simulink model "model_chirp_control_conMR_Bingham"  (R2016a)
settings: Solver=ode4  StartTime=0.0  StopTime=t_final2  FixedStep=tsam  RelTol=1e-3
values from neighbouring files (symbols this model uses):
  I1 = 0.01    [Run_MdE_Research_Report_con_MR_damper.m]
  kt = ((2*pi*ft)^2)*mt    [Run_MdE_Research_Report.m]    (also in Run_MdE_Research_Report_con_MR_damper.m; my_script.m)
  mt = mu*m1    (= 0.02)    [Run_MdE_Research_Report.m]    (also in Run_MdE_Research_Report_con_MR_damper.m = 40; my_script.m)
  sat = 50    [Run_MdE_Research_Report_con_MR_damper.m]
undefined symbols (not defined in the file or in its folder): D_Gs, N_Gs, ndata2, t_final2, tsam
libraries: simulink x1
settings Model: Creator=user  LastModifiedBy=usuario
settings DataIOCC: LimitDataPoints=on  SaveFormat=Array  SignalLoggingSaveFormat=ModelDataLogs  SignalLoggingName=sigsOut
settings OptimizationCC: InitFltsAndDblsToZero=on
settings DebuggingCC: SaveWithParameterizedLinksMsg=none  UnderspecifiedInitializationDetection=Classic  MergeDetectMultiDrivingBlocksExec=none  SignalResolutionControl=TryResolveAllWithWarning  MultiTaskDSMMsg=warning  MultiTaskCondExecSysMsg=none  FcnCallInpInsideContextMsg=EnableAllAsWarning
settings HardwareCC: ProdBitPerPointer=32  ProdLargestAtomicFloat=None  ProdIntDivRoundTo=Undefined  ProdEndianess=Unspecified  ProdWordSize=32  ProdHWDeviceType=32-bit Generic  TargetBitPerPointer=64  TargetLongLongMode=on  TargetIntDivRoundTo=Zero  TargetEndianess=LittleEndian  TargetWordSize=64  TargetHWDeviceType=MATLAB Host  ProdEqTarget=off
settings ModelReferenceCC: PropagateSignalLabelsOutOfModel=off
settings GRTTargetCC: TargetFcnLib=ansi_tfl_tmw.mat  CombineOutputUpdateFcns=off  GRTInterface=on
settings ConfigComp: CovModelRefEnable=Off  CovSFcnEnable=off

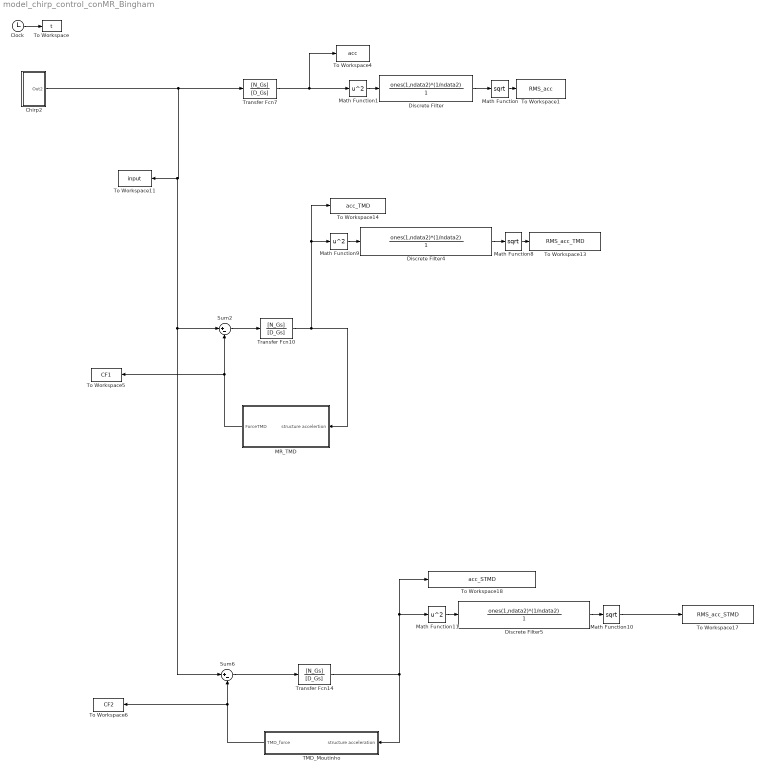
== system model_chirp_control_conMR_Bingham ==
  Chirp2 : Subsystem
  Clock : Clock
  Discrete Filter : DiscreteFilter  Numerator=ones(1,ndata2)*(1/ndata2)  Denominator=1  SampleTime=tsam
  Discrete Filter4 : DiscreteFilter  Numerator=ones(1,ndata2)*(1/ndata2)  Denominator=1  SampleTime=tsam
  Discrete Filter5 : DiscreteFilter  Numerator=ones(1,ndata2)*(1/ndata2)  Denominator=1  SampleTime=tsam
  MR_TMD : Subsystem
  Math Function : Math  Operator=sqrt  SampleTime=tsam  SaturateOnIntegerOverflow=on
  Math Function1 : Math  Operator=square  SampleTime=tsam  SaturateOnIntegerOverflow=on
  Math Function10 : Math  Operator=sqrt  SampleTime=tsam  SaturateOnIntegerOverflow=on
  Math Function11 : Math  Operator=square  SampleTime=tsam  SaturateOnIntegerOverflow=on
  Math Function8 : Math  Operator=sqrt  SampleTime=tsam  SaturateOnIntegerOverflow=on
  Math Function9 : Math  Operator=square  SampleTime=tsam  SaturateOnIntegerOverflow=on
  Sum2 : Sum  Inputs=|+-
  Sum6 : Sum  Inputs=|+-
  TMD_Moutinho : Subsystem
  To Workspace : ToWorkspace  VariableName=t  SampleTime=tsam
  To Workspace1 : ToWorkspace  VariableName=RMS_acc  SampleTime=tsam
  To Workspace11 : ToWorkspace  VariableName=input  SampleTime=tsam
  To Workspace13 : ToWorkspace  VariableName=RMS_acc_TMD  SampleTime=tsam
  To Workspace14 : ToWorkspace  VariableName=acc_TMD  SampleTime=tsam
  To Workspace17 : ToWorkspace  VariableName=RMS_acc_STMD  SampleTime=tsam
  To Workspace18 : ToWorkspace  VariableName=acc_STMD  SampleTime=tsam
  To Workspace4 : ToWorkspace  VariableName=acc  SampleTime=tsam
  To Workspace5 : ToWorkspace  VariableName=CF1  SampleTime=tsam
  To Workspace6 : ToWorkspace  VariableName=CF2  SampleTime=tsam
  Transfer Fcn10 : TransferFcn  Numerator=[N_Gs]  Denominator=[D_Gs]
  Transfer Fcn14 : TransferFcn  Numerator=[N_Gs]  Denominator=[D_Gs]
  Transfer Fcn7 : TransferFcn  Numerator=[N_Gs]  Denominator=[D_Gs]
  wires:
  Clock/1 -> To Workspace/1
  Math Function1/1 -> Discrete Filter/1
  Discrete Filter/1 -> Math Function/1
  Math Function/1 -> To Workspace1/1
  Sum2/1 -> Transfer Fcn10/1
  Math Function9/1 -> Discrete Filter4/1
  Discrete Filter4/1 -> Math Function8/1
  Math Function8/1 -> To Workspace13/1
  MR_TMD/1(ForceTMD) -> Sum2/2, To Workspace5/1
  Transfer Fcn7/1 -> Math Function1/1, To Workspace4/1
  Transfer Fcn10/1 -> MR_TMD/1(structure accelertion), To Workspace14/1, Math Function9/1
  Math Function11/1 -> Discrete Filter5/1
  Discrete Filter5/1 -> Math Function10/1
  Math Function10/1 -> To Workspace17/1
  Sum6/1 -> Transfer Fcn14/1
  Chirp2/1(Out2) -> Sum2/1, Sum6/1, To Workspace11/1, Transfer Fcn7/1
  Transfer Fcn14/1 -> TMD_Moutinho/1(structure acceleration), Math Function11/1, To Workspace18/1
  TMD_Moutinho/1(TMD_force) -> To Workspace6/1, Sum6/2

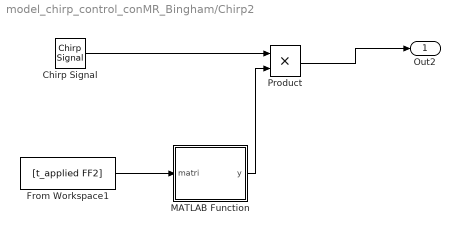
== system model_chirp_control_conMR_Bingham/Chirp2 ==
  Chirp Signal : simulink/Sources/Chirp Signal  f1=f_ini  T=t_final2  f2=f_fin
  From Workspace1 : FromWorkspace  VariableName=[t_applied FF2]  SampleTime=tsam
  MATLAB Function : MATLAB Function  TreatAsAtomicUnit=on
  Product : Product
  Out2 : Outport
  wires:
  Chirp Signal/1 -> Product/1
  MATLAB Function/1(y) -> Product/2
  Product/1 -> Out2/1
  From Workspace1/1 -> MATLAB Function/1(matri)

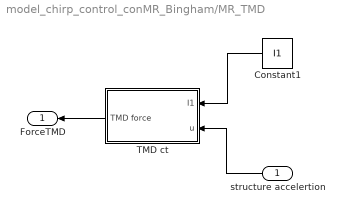
== system model_chirp_control_conMR_Bingham/MR_TMD ==
  structure accelertion : Inport
  Constant1 : Constant  Value=I1
  TMD ct : Subsystem
  ForceTMD : Outport
  wires:
  TMD ct/1(TMD force) -> ForceTMD/1
  structure accelertion/1 -> TMD ct/2(u)
  Constant1/1 -> TMD ct/1(I1)

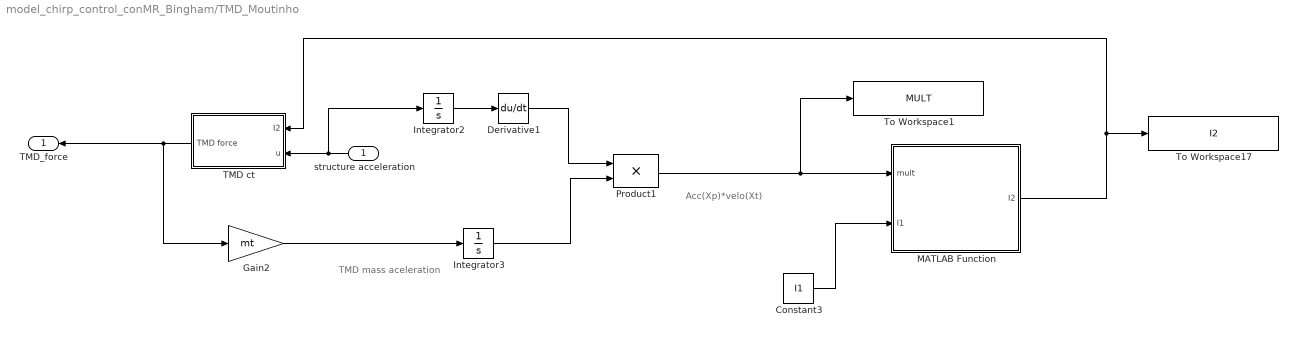
== system model_chirp_control_conMR_Bingham/TMD_Moutinho ==
  note: TMD mass
      | aceleration
  note: Acc(Xp)*velo(Xt)
  structure acceleration : Inport
  Constant3 : Constant  Value=I1
  Derivative1 : Derivative
  Gain2 : Gain  Gain=mt
  Integrator2 : Integrator
  Integrator3 : Integrator
  MATLAB Function : MATLAB Function  TreatAsAtomicUnit=on
  Product1 : Product  OutDataTypeStr=double  SaturateOnIntegerOverflow=on
  TMD ct : Subsystem
  To Workspace1 : ToWorkspace  VariableName=MULT  SampleTime=tsam
  To Workspace17 : ToWorkspace  VariableName=I2  SampleTime=tsam
  TMD_force : Outport
  wires:
  TMD ct/1(TMD force) -> Gain2/1, TMD_force/1
  Integrator3/1 -> Product1/2
  Product1/1 -> To Workspace1/1, MATLAB Function/1(mult)
  MATLAB Function/1(I2) -> TMD ct/1(I2), To Workspace17/1
  structure acceleration/1 -> TMD ct/2(u), Integrator2/1
  Integrator2/1 -> Derivative1/1
  Derivative1/1 -> Product1/1
  Gain2/1 -> Integrator3/1
  Constant3/1 -> MATLAB Function/2(I1)

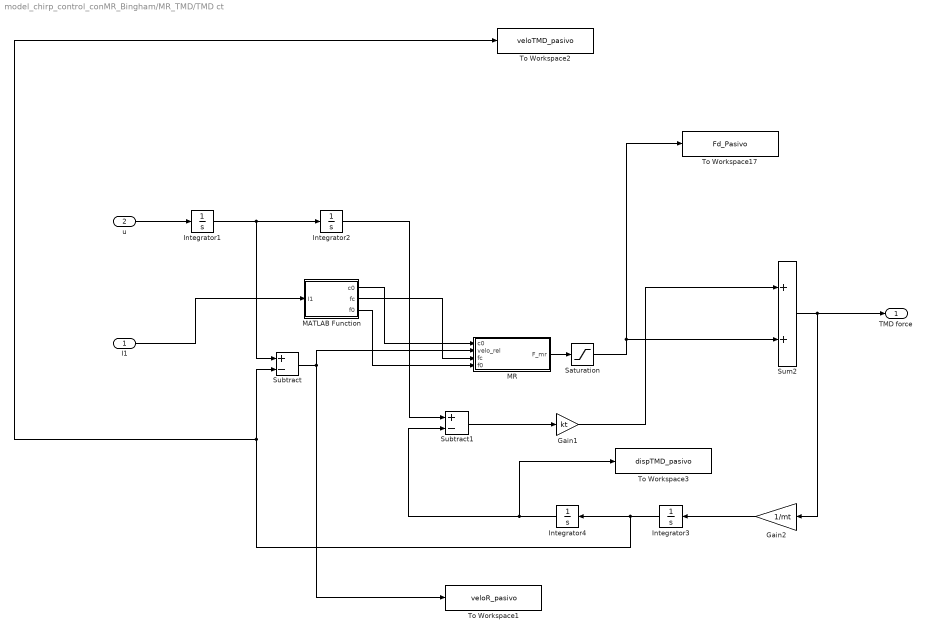
== system model_chirp_control_conMR_Bingham/MR_TMD/TMD ct ==
  I1 : Inport
  u : Inport  Port=2
  Gain1 : Gain  Gain=kt
  Gain2 : Gain  Gain=1/mt
  Integrator{1..4} (4 alike) : Integrator
  MATLAB Function : MATLAB Function  TreatAsAtomicUnit=on
  MR : Subsystem
  Saturation : Saturate  UpperLimit=sat  LowerLimit=-sat
  Subtract : Sum  Inputs=+-
  Subtract1 : Sum  Inputs=+-
  Sum2 : Sum
  To Workspace1 : ToWorkspace  VariableName=veloR_pasivo  SampleTime=tsam
  To Workspace17 : ToWorkspace  VariableName=Fd_Pasivo  SampleTime=tsam
  To Workspace2 : ToWorkspace  VariableName=veloTMD_pasivo  SampleTime=tsam
  To Workspace3 : ToWorkspace  VariableName=dispTMD_pasivo  SampleTime=tsam
  TMD force : Outport
  wires:
  Integrator1/1 -> Subtract/1, Integrator2/1
  u/1 -> Integrator1/1
  I1/1 -> MATLAB Function/1(I1)
  Integrator3/1 -> Integrator4/1, To Workspace2/1, Subtract/2
  Subtract/1 -> MR/2(velo_rel), To Workspace1/1
  Gain2/1 -> Integrator3/1
  Integrator4/1 -> To Workspace3/1, Subtract1/2
  Integrator2/1 -> Subtract1/1
  Subtract1/1 -> Gain1/1
  Gain1/1 -> Sum2/1
  Sum2/1 -> Gain2/1, TMD force/1
  MR/1(F_mr) -> Saturation/1
  MATLAB Function/1(c0) -> MR/1(c0)
  MATLAB Function/2(fc) -> MR/3("fc ")
  MATLAB Function/3(f0) -> MR/4(f0)
  Saturation/1 -> To Workspace17/1, Sum2/2

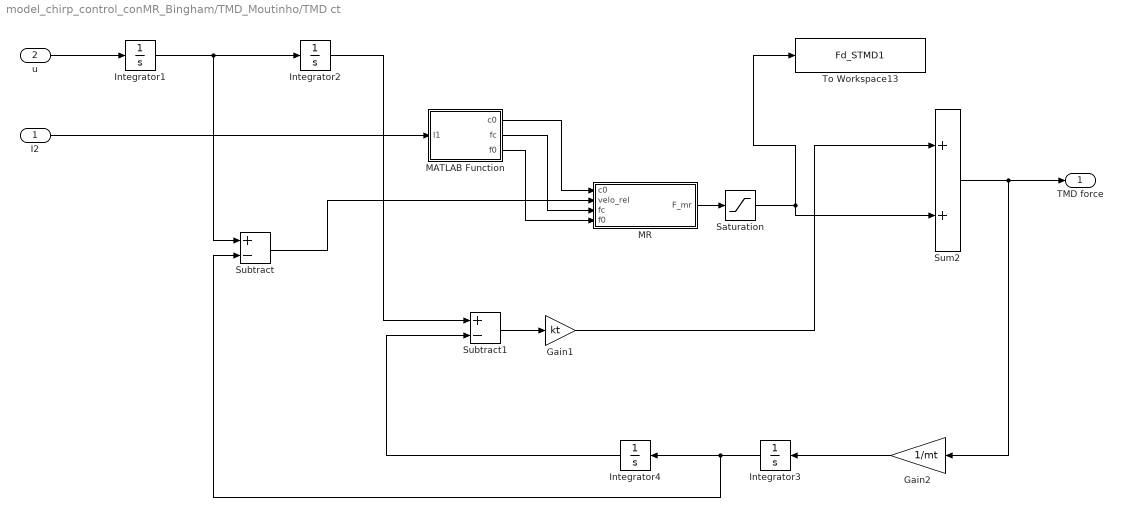
== system model_chirp_control_conMR_Bingham/TMD_Moutinho/TMD ct ==
  I2 : Inport
  u : Inport  Port=2
  Gain1 : Gain  Gain=kt
  Gain2 : Gain  Gain=1/mt
  Integrator{1..4} (4 alike) : Integrator
  MATLAB Function : MATLAB Function  TreatAsAtomicUnit=on
  MR : Subsystem
  Saturation : Saturate  UpperLimit=sat  LowerLimit=-sat
  Subtract : Sum  Inputs=+-
  Subtract1 : Sum  Inputs=+-
  Sum2 : Sum
  To Workspace13 : ToWorkspace  VariableName=Fd_STMD1  SampleTime=tsam
  TMD force : Outport
  wires:
  Integrator1/1 -> Subtract/1, Integrator2/1
  u/1 -> Integrator1/1
  Integrator3/1 -> Integrator4/1, Subtract/2
  Gain2/1 -> Integrator3/1
  Integrator4/1 -> Subtract1/2
  Integrator2/1 -> Subtract1/1
  Subtract1/1 -> Gain1/1
  Gain1/1 -> Sum2/1
  Sum2/1 -> Gain2/1, TMD force/1
  I2/1 -> MATLAB Function/1(I1)
  Subtract/1 -> MR/2(velo_rel)
  MATLAB Function/1(c0) -> MR/1(c0)
  MATLAB Function/2(fc) -> MR/3("fc ")
  MR/1(F_mr) -> Saturation/1
  Saturation/1 -> Sum2/2, To Workspace13/1
  MATLAB Function/3(f0) -> MR/4(f0)

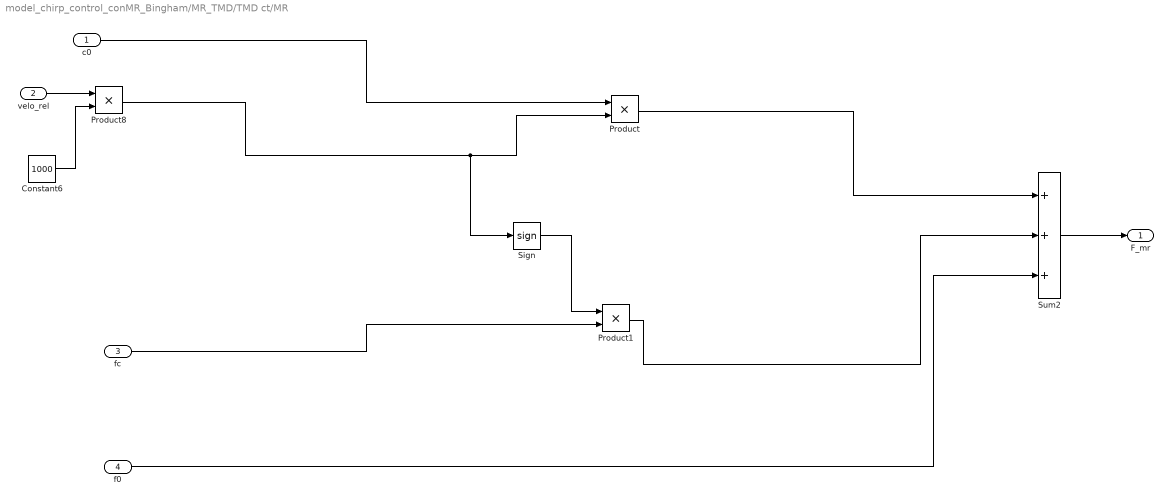
== system model_chirp_control_conMR_Bingham/MR_TMD/TMD ct/MR ==
  c0 : Inport
  velo_rel : Inport  Port=2
  "fc " : Inport  Port=3
  f0 : Inport  Port=4
  Constant6 : Constant  Value=1000
  Product : Product
  Product1 : Product
  Product8 : Product
  Sign : Signum
  Sum2 : Sum  Inputs=+++
  F_mr : Outport
  wires:
  velo_rel/1 -> Product8/1
  Constant6/1 -> Product8/2
  c0/1 -> Product/1
  Sum2/1 -> F_mr/1
  Product1/1 -> Sum2/2
  Product/1 -> Sum2/1
  Product8/1 -> Sign/1, Product/2
  "fc "/1 -> Product1/2
  Sign/1 -> Product1/1
  f0/1 -> Sum2/3

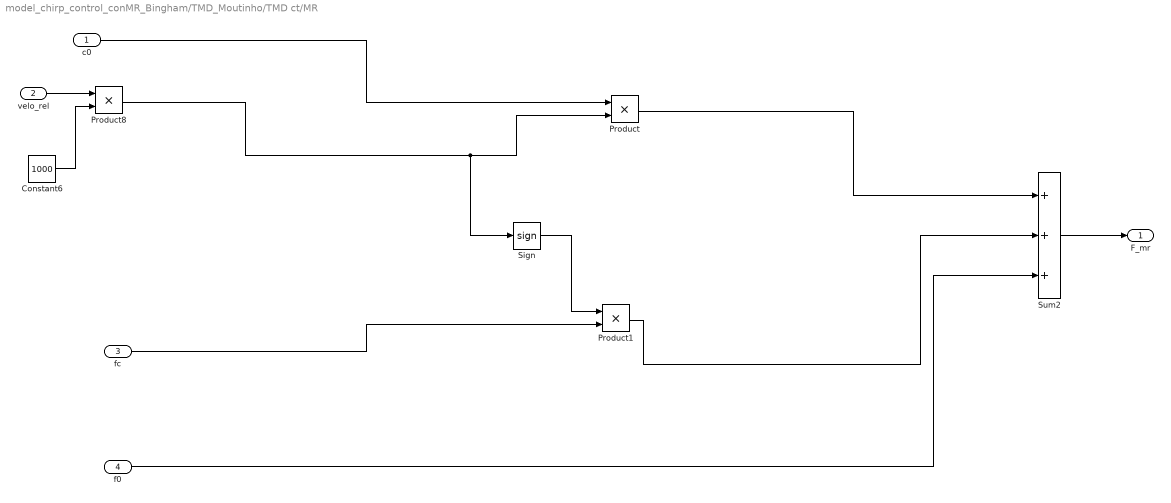
== system model_chirp_control_conMR_Bingham/TMD_Moutinho/TMD ct/MR ==
  c0 : Inport
  velo_rel : Inport  Port=2
  "fc " : Inport  Port=3
  f0 : Inport  Port=4
  Constant6 : Constant  Value=1000
  Product : Product
  Product1 : Product
  Product8 : Product
  Sign : Signum
  Sum2 : Sum  Inputs=+++
  F_mr : Outport
  wires:
  velo_rel/1 -> Product8/1
  Constant6/1 -> Product8/2
  c0/1 -> Product/1
  Sum2/1 -> F_mr/1
  Product1/1 -> Sum2/2
  Product/1 -> Sum2/1
  Product8/1 -> Sign/1, Product/2
  "fc "/1 -> Product1/2
  Sign/1 -> Product1/1
  f0/1 -> Sum2/3

== matlab function model_chirp_control_conMR_Bingham/MR_TMD/TMD ct/MATLAB Function ==
  data: I1 input; c0 output; fc output; f0 output
function [c0,fc,f0] = fcn(I1)
f0 = 0;
c0 = -0.079*I1^3 - 0.133*I1^2 + 0.184*I1 + 0.004;
fc = -85.19*I1^3 + 75.67*I1^2 + 24.95*I1 +0.14;

== matlab function model_chirp_control_conMR_Bingham/Chirp2/MATLAB Function ==
  data: y output; matri input
function y = fcn(matri)

% time = matri(:,1);
% force = matri(:,2);
% 
% pos = find( u>= time);
% pos2 = pos(1);


y = matri; %force(pos);

== matlab function model_chirp_control_conMR_Bingham/TMD_Moutinho/MATLAB Function ==
  data: mult input; I2 output; I1 input
function I2 = fcn(mult,I1)

if mult <= 0
    I2 = I1;
else
    I2 = 0.5;
end

== matlab function model_chirp_control_conMR_Bingham/TMD_Moutinho/TMD ct/MATLAB Function ==
  data: I1 input; c0 output; fc output; f0 output
function [c0,fc,f0] = fcn(I1)
f0 = 0;
c0 = -0.079*I1^3 - 0.133*I1^2 + 0.184*I1 + 0.004;
fc = -85.19*I1^3 + 75.67*I1^2 + 24.95*I1 +0.14;
